simulink model "bot_sim"  (R2026a)
settings: Solver=FixedStepAuto  StopTime=tspan  FixedStep=dt_sim
undefined symbols (not defined in the file): dt_control, dt_data, dt_sim, P, scene_struct, X0
libraries: ros2lib x3
settings Model: Creator=koryh  LastModifiedBy=matthewlin

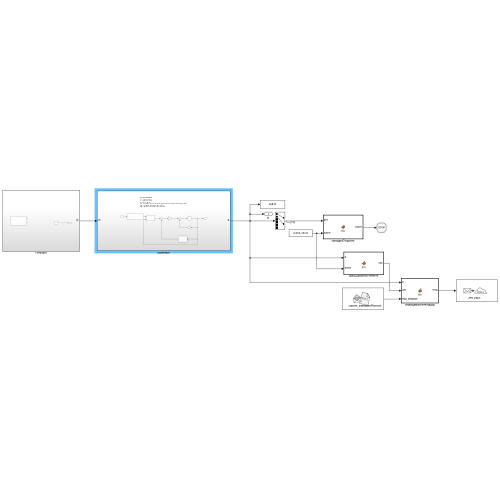
[thumbnail: Simulink's stored preview of the top-level diagram]
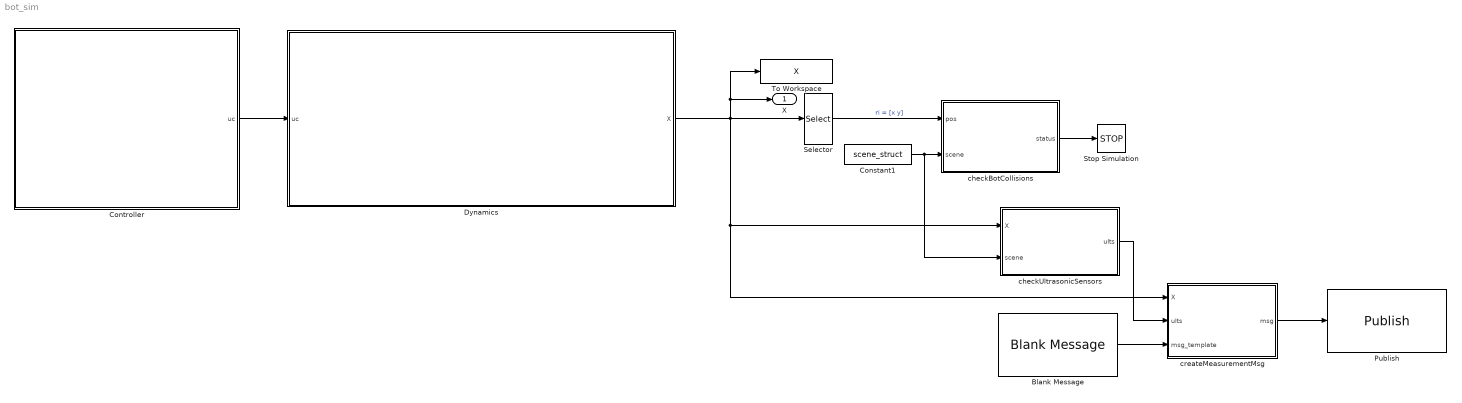
== system bot_sim ==
  Blank Message : ros2lib/Blank Message  messageClass=Message  entityType=custom_interfaces/Sensors  messageType=custom_interfaces/Sensors  SampleTime=inf
  Constant1 : Constant  Value=scene_struct  OutDataTypeStr=Bus: scene_bus
  Controller : Subsystem
  Dynamics : Subsystem
  Publish : ros2lib/Publish  topicSource=Specify your own  topic=/my_topic  messageType=custom_interfaces/Sensors  QOSHistory=Keep last  QOSDepth=10  QOSReliability=Reliable  QOSDurability=Volatile  QOSDeadline=Inf  QOSLifespan=Inf  QOSLiveliness=Automatic  QOSLeaseDuration=Inf  QOSAvoidROSNamespaceConventions=off
  Selector : Selector  InputPortWidth=6  IndexOptions=Index vector (dialog)  Indices=[1 2]  OutputSizes=1
  Stop Simulation : Stop
  To Workspace : ToWorkspace  VariableName=X  SaveFormat=Timeseries  SampleTime=dt_data
  checkBotCollisions : MATLAB Function  TreatAsAtomicUnit=on
  checkUltrasonicSensors : MATLAB Function  TreatAsAtomicUnit=on
  createMeasurementMsg : MATLAB Function  TreatAsAtomicUnit=on
  X : Outport
  wires:
  Dynamics/1(X) -> Selector/1, X/1, To Workspace/1, checkUltrasonicSensors/1(X), createMeasurementMsg/1(X)
  Selector/1 -> checkBotCollisions/1(pos)  "ri = [x y]"
  checkBotCollisions/1(status) -> Stop Simulation/1
  Constant1/1 -> checkUltrasonicSensors/2(scene), checkBotCollisions/2(scene)
  checkUltrasonicSensors/1(ults) -> createMeasurementMsg/2(ults)
  Blank Message/1 -> createMeasurementMsg/3(msg_template)
  createMeasurementMsg/1(msg) -> Publish/1
  Controller/1(uc) -> Dynamics/1(uc)

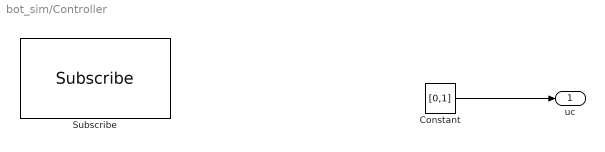
== system bot_sim/Controller ==
  Constant : Constant  Value=[0,1]
  Subscribe : ros2lib/Subscribe  topicSource=Specify your own  topic=/my_topic  messageType=custom_interfaces/Sensors  sampleTime=dt_control  QOSHistory=Keep last  QOSDepth=10  QOSReliability=Reliable  QOSDurability=Volatile  QOSDeadline=Inf  QOSLifespan=Inf  QOSLiveliness=Automatic  QOSLeaseDuration=Inf  QOSAvoidROSNamespaceConventions=off
  uc : Outport
  wires:
  Constant/1 -> uc/1

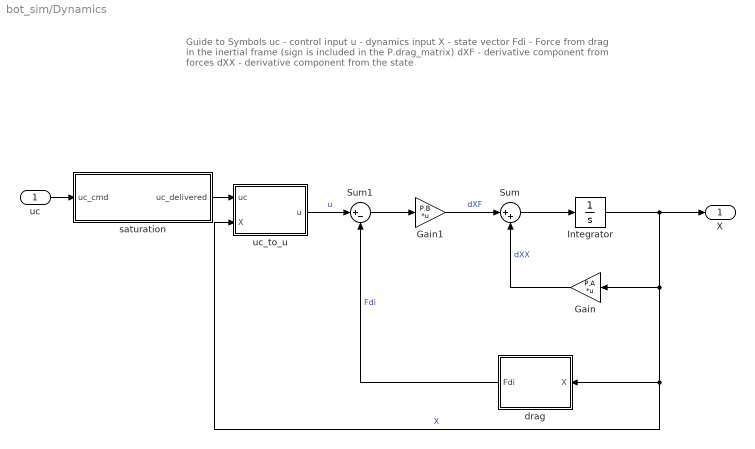
== system bot_sim/Dynamics ==
  note: Guide to Symbols
      | uc - control input
      | u - dynamics input
      | X - state vector
      | Fdi - Force from drag in the inertial frame (sign is included in the P.drag_matrix)
      | dXF - derivative component from forces
      | dXX - derivative component from the state
  uc : Inport  SampleTime=dt_sim
  Gain : Gain  Gain=P.A  Multiplication=Matrix(K*u)
  Gain1 : Gain  Gain=P.B  Multiplication=Matrix(K*u)
  Integrator : Integrator  InitialCondition=X0
  Sum : Sum  Inputs=|++
  Sum1 : Sum  Inputs=|+-
  drag : MATLAB Function  TreatAsAtomicUnit=on
  saturation : MATLAB Function  TreatAsAtomicUnit=on
  uc_to_u : MATLAB Function  TreatAsAtomicUnit=on
  X : Outport  SampleTime=dt_control
  wires:
  Integrator/1 -> X/1, Gain/1, drag/1(X), uc_to_u/2(X)  "X"
  Gain1/1 -> Sum/1  "dXF"
  Gain/1 -> Sum/2  "dXX"
  uc/1 -> saturation/1(uc_cmd)
  uc_to_u/1(u) -> Sum1/1  "u"
  drag/1(Fdi) -> Sum1/2  "Fdi"
  Sum1/1 -> Gain1/1
  Sum/1 -> Integrator/1
  saturation/1(uc_delivered) -> uc_to_u/1(uc)

== matlab function bot_sim/checkUltrasonicSensors ==
  data: X input; ults output; scene input
function ults = fcn(X, scene)

ults = checkUltrasonicSensors(X, scene);

== matlab function bot_sim/Dynamics/uc_to_u ==
  data: uc input; u output; X input
function u = fcn(uc, X)
%{
Convert the control input uc = [Fbx, M] into the dynamics input u = [Fix,
Fiy, M] so the dynamics model can remain linear.
%}

%Unpack yaw from the dynamics
psi = X(5);

u = [cos(psi) 0;sin(psi) 0;0 1]*uc;

== matlab function bot_sim/Dynamics/drag ==
  data: Fdi output; X input; P parameter
function Fdi = fcn(X,P)
%{
Calculates the drag force and moment and returns the value in the inertial
frame.
%}

%Unpack yaw and velocity from the dynamics
psi = X(5); %yaw
dpsi = X(6); %yaw rate

%Unpack the inertial frame velocity
vi = [X(3);X(4)];

%Rotation matrices
Cbi = [cos(psi) sin(psi); -sin(psi) cos(psi)]; %inertial to body
Cib = Cbi'; %body to inertial

%Compute the velocity in the body frame
vb = Cbi*vi;

%Calculate the linear and rotational drag in the body frame
Fdb = P.drag_matrix*[vb;dpsi];

%Convert the linear portion back to the inertial frame
Fdi_lin = Cib*[Fdb(1);Fdb(2)];

%repack
Fdi = [Fdi_lin;Fdb(3)]; %yaw drag is the same in both frames

== matlab function bot_sim/Dynamics/saturation ==
  data: uc_cmd input; uc_delivered output
function uc_delivered = fcn(uc_cmd)

uc_delivered = zeros(2,1);

%constrain to max values
uc_delivered(1) = min(max(uc_cmd(1),2.5),-2.5);
uc_delivered(2) = min(max(uc_cmd(2),2),-2);

== matlab function bot_sim/createMeasurementMsg ==
  data: X input; msg output Bus: SL_Bus_custom_interfaces_Sensors; ults input; msg_template input
function msg = fcn(X, ults, msg_template)

msg = msg_template;
msg.x = X(1);
msg.y = X(2);
msg.yaw = X(5);
msg.d1 = ults(1);
msg.d2 = ults(2);
msg.d3 = ults(3);

== matlab function bot_sim/checkBotCollisions ==
  data: pos input; status output; scene input
function status  = fcn(pos, scene)

[status, ~] = checkBotCollision(pos', scene);
